simulink model "ThreeSinglePhaseDiodeRectifierSchematic"  (R2018a)
settings: Solver=VariableStepAuto  StartTime=0.0  StopTime=0.1  RelTol=1e-3
libraries: powerlib x32
settings Model: Creator=mertelmas  LastModifiedBy=mertelmas

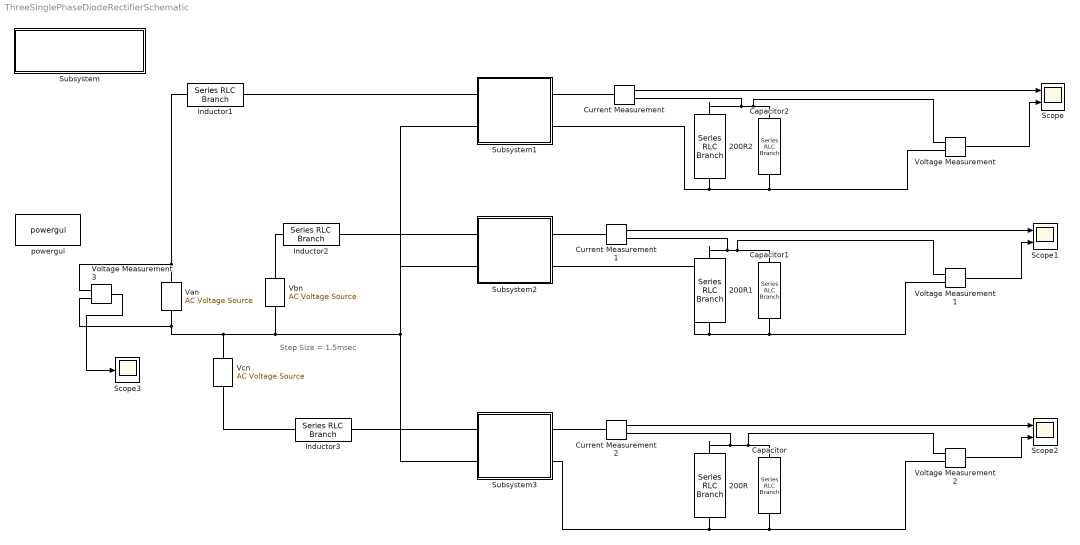
== system ThreeSinglePhaseDiodeRectifierSchematic ==
  note: Step Size = 1.5msec
  200R : powerlib/Elements/Series RLC Branch  LConnTagsString=__new0  RConnTagsString=__new0  BranchType=R  Resistance=200  Inductance=1e-3  SetiL0=off  InitialCurrent=0  Capacitance=1e-6  Setx0=off  InitialVoltage=0  Measurements=None
  200R1 : powerlib/Elements/Series RLC Branch  LConnTagsString=__new0  RConnTagsString=__new0  BranchType=R  Resistance=200  Inductance=1e-3  SetiL0=off  InitialCurrent=0  Capacitance=1e-6  Setx0=off  InitialVoltage=0  Measurements=None
  200R2 : powerlib/Elements/Series RLC Branch  LConnTagsString=__new0  RConnTagsString=__new0  BranchType=R  Resistance=200  Inductance=1e-3  SetiL0=off  InitialCurrent=0  Capacitance=1e-6  Setx0=off  InitialVoltage=0  Measurements=None
  Capacitor : powerlib/Elements/Series RLC Branch  LConnTagsString=__new0  RConnTagsString=__new0  BranchType=C  Resistance=1  Inductance=1e-3  SetiL0=off  InitialCurrent=0  Capacitance=47e-5  Setx0=off  InitialVoltage=0  Measurements=None
  Capacitor1 : powerlib/Elements/Series RLC Branch  LConnTagsString=__new0  RConnTagsString=__new0  BranchType=C  Resistance=1  Inductance=1e-3  SetiL0=off  InitialCurrent=0  Capacitance=47e-5  Setx0=off  InitialVoltage=0  Measurements=None
  Capacitor2 : powerlib/Elements/Series RLC Branch  LConnTagsString=__new0  RConnTagsString=__new0  BranchType=C  Resistance=1  Inductance=1e-3  SetiL0=off  InitialCurrent=0  Capacitance=47e-5  Setx0=off  InitialVoltage=0  Measurements=None
  Current Measurement : powerlib/Measurements/Current Measurement  PhasorSimulation=off  OutputType=Complex  PSBequivalent=0
  Current Measurement1 : powerlib/Measurements/Current Measurement  PhasorSimulation=off  OutputType=Complex  PSBequivalent=0
  Current Measurement2 : powerlib/Measurements/Current Measurement  PhasorSimulation=off  OutputType=Complex  PSBequivalent=0
  Inductor1 : powerlib/Elements/Series RLC Branch  LConnTagsString=__new0  RConnTagsString=__new0  BranchType=L  Resistance=1  Inductance=6e-4  SetiL0=off  InitialCurrent=0  Capacitance=1e-6  Setx0=off  InitialVoltage=0  Measurements=None
  Inductor2 : powerlib/Elements/Series RLC Branch  LConnTagsString=__new0  RConnTagsString=__new0  BranchType=L  Resistance=1  Inductance=6e-4  SetiL0=off  InitialCurrent=0  Capacitance=1e-6  Setx0=off  InitialVoltage=0  Measurements=None
  Inductor3 : powerlib/Elements/Series RLC Branch  LConnTagsString=__new0  RConnTagsString=__new0  BranchType=L  Resistance=1  Inductance=6e-4  SetiL0=off  InitialCurrent=0  Capacitance=1e-6  Setx0=off  InitialVoltage=0  Measurements=None
  Scope : Scope  NumInputPorts=2
  Scope1 : Scope  NumInputPorts=2
  Scope2 : Scope  NumInputPorts=2
  Scope3 : Scope
  Subsystem : Subsystem
      settings: OpenFcn=open_system('power_new_palette')
      mask Display: disp(sprintf('Open Simscape Power Systems\n(Specialized Technology)\nPalette Library'));
  Subsystem1 : Subsystem
  Subsystem2 : Subsystem
  Subsystem3 : Subsystem
  Van : powerlib/Electrical Sources/AC Voltage Source  Amplitude=325.27  Phase=0  Frequency=50  SampleTime=0  Measurements=None  BusType=swing  Pref=10e3  Qref=0  Qmin=-inf  Qmax=+inf
  Vbn : powerlib/Electrical Sources/AC Voltage Source  Amplitude=325.27  Phase=120  Frequency=50  SampleTime=0  Measurements=None  BusType=swing  Pref=10e3  Qref=0  Qmin=-inf  Qmax=+inf
  Vcn : powerlib/Electrical Sources/AC Voltage Source  Amplitude=325.27  Phase=240  Frequency=50  SampleTime=0  Measurements=None  BusType=swing  Pref=10e3  Qref=0  Qmin=-inf  Qmax=+inf
  Voltage Measurement{,1..3} (4 alike) : powerlib/Measurements/Voltage Measurement  PhasorSimulation=off  OutputType=Complex  PSBequivalent=0
  powergui : powerlib/powergui  Priority=1  SimulationMode=Continuous  SampleTime=50e-6  frequency=60  Iterations=50  frequencyindice=50  Pbase=100e6  ErrMax=1e-4  UnitsV=kV  UnitsW=MW  buscounter=0  FunctionMessages=off  echomessages=off  EnableUseOfTLC=off  CurrentSourceSwitches=off  DisableSnubberDevices=off  DisableRonSwitches=off  DisableVfSwitches=off  DisplayEquations=off  SolverType=Tustin/Backward Euler (TBE)  Interpol=off  ExternalGateDelay=off  methode=off  Ts=100  x0status=blocks  SPID=on  SwTol=0  HookPort=off  RestoreLinks=warning  ResistiveCurrentMeasurement=off  Frange=[0:2:500]  Ylog=off  Xlog=on  ShowGrid=off  save=off  variable=ZData  structure=0  ZoomFFT=off  StartTime=0.0  cycles=1  DisplayStyle=1  fundamental=60  FreqAxis=off  MaxFrequency=1000  frequencyindicesteady=1  RmsSteady=1  display=off
  wires:
  Current Measurement/1 -> Scope/1
  Current Measurement1/1 -> Scope1/1
  Current Measurement2/1 -> Scope2/1
  Voltage Measurement2/1 -> Scope2/2
  Voltage Measurement1/1 -> Scope1/2
  Voltage Measurement/1 -> Scope/2
  Voltage Measurement3/1 -> Scope3/1
  connections:
  Van/LConn1 -- Voltage Measurement3/LConn2 -- Vcn/LConn1 -- Subsystem1/LConn2 -- Subsystem2/LConn2 -- Subsystem3/LConn2 -- Vbn/LConn1
  Vcn/RConn1 -- Inductor3/LConn1
  Inductor1/LConn1 -- Voltage Measurement3/LConn1 -- Van/RConn1
  Vbn/RConn1 -- Inductor2/LConn1
  200R/LConn1 -- Current Measurement2/RConn1 -- Voltage Measurement2/LConn1 -- Capacitor/LConn1
  200R/RConn1 -- Voltage Measurement2/LConn2 -- Capacitor/RConn1 -- Subsystem3/RConn2
  200R1/LConn1 -- Current Measurement1/RConn1 -- Voltage Measurement1/LConn1 -- Capacitor1/LConn1
  200R1/RConn1 -- Voltage Measurement1/LConn2 -- Capacitor1/RConn1 -- Subsystem2/RConn2
  200R2/LConn1 -- Current Measurement/RConn1 -- Voltage Measurement/LConn1 -- Capacitor2/LConn1
  Inductor1/RConn1 -- Subsystem1/LConn1
  Inductor2/RConn1 -- Subsystem2/LConn1
  Subsystem3/LConn1 -- Inductor3/RConn1
  200R2/RConn1 -- Voltage Measurement/LConn2 -- Capacitor2/RConn1 -- Subsystem1/RConn2
  Current Measurement/LConn1 -- Subsystem1/RConn1
  Subsystem2/RConn1 -- Current Measurement1/LConn1
  Subsystem3/RConn1 -- Current Measurement2/LConn1

== system ThreeSinglePhaseDiodeRectifierSchematic/Subsystem ==

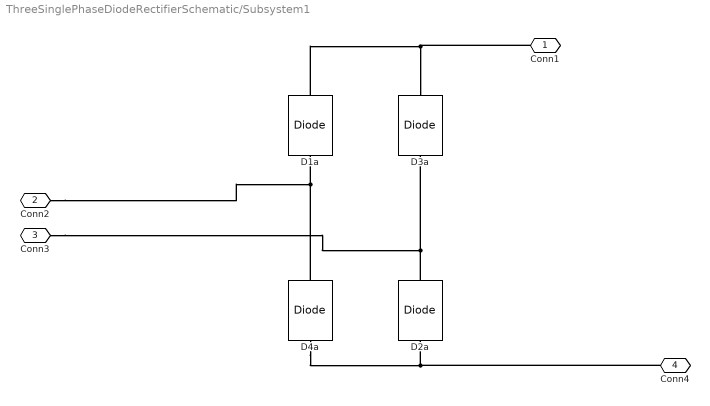
== system ThreeSinglePhaseDiodeRectifierSchematic/Subsystem1 ==
  D1a : powerlib/Power Electronics/Diode  Ron=0.001  Lon=0  Vf=0.8  IC=0  UseSnubber=0  Rs=500  Cs=250e-9  Measurements=off
  D2a : powerlib/Power Electronics/Diode  Ron=0.001  Lon=0  Vf=0.8  IC=0  UseSnubber=0  Rs=500  Cs=250e-9  Measurements=off
  D3a : powerlib/Power Electronics/Diode  Ron=0.001  Lon=0  Vf=0.8  IC=0  UseSnubber=0  Rs=500  Cs=250e-9  Measurements=off
  D4a : powerlib/Power Electronics/Diode  Ron=0.001  Lon=0  Vf=0.8  IC=0  UseSnubber=0  Rs=500  Cs=250e-9  Measurements=off
  Conn1 : PMIOPort  Side=Right
  Conn2 : PMIOPort  Port=2  Side=Left
  Conn3 : PMIOPort  Port=3  Side=Left
  Conn4 : PMIOPort  Port=4  Side=Right
  connections:
  D1a/RConn1 -- D3a/RConn1 -- Conn1/RConn1
  D2a/RConn1 -- D3a/LConn1 -- Conn3/RConn1
  D4a/LConn1 -- D2a/LConn1 -- Conn4/RConn1
  D4a/RConn1 -- D1a/LConn1 -- Conn2/RConn1

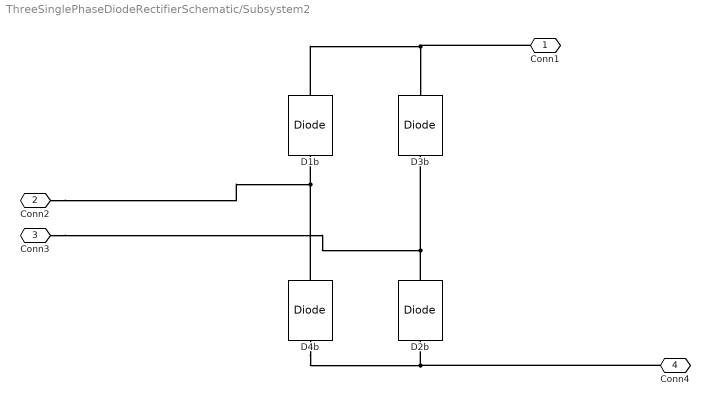
== system ThreeSinglePhaseDiodeRectifierSchematic/Subsystem2 ==
  D1b : powerlib/Power Electronics/Diode  Ron=0.001  Lon=0  Vf=0.8  IC=0  UseSnubber=0  Rs=500  Cs=250e-9  Measurements=off
  D2b : powerlib/Power Electronics/Diode  Ron=0.001  Lon=0  Vf=0.8  IC=0  UseSnubber=0  Rs=500  Cs=250e-9  Measurements=off
  D3b : powerlib/Power Electronics/Diode  Ron=0.001  Lon=0  Vf=0.8  IC=0  UseSnubber=0  Rs=500  Cs=250e-9  Measurements=off
  D4b : powerlib/Power Electronics/Diode  Ron=0.001  Lon=0  Vf=0.8  IC=0  UseSnubber=0  Rs=500  Cs=250e-9  Measurements=off
  Conn1 : PMIOPort  Side=Right
  Conn2 : PMIOPort  Port=2  Side=Left
  Conn3 : PMIOPort  Port=3  Side=Left
  Conn4 : PMIOPort  Port=4  Side=Right
  connections:
  D1b/RConn1 -- D3b/RConn1 -- Conn1/RConn1
  D2b/RConn1 -- D3b/LConn1 -- Conn3/RConn1
  D4b/LConn1 -- D2b/LConn1 -- Conn4/RConn1
  D4b/RConn1 -- D1b/LConn1 -- Conn2/RConn1

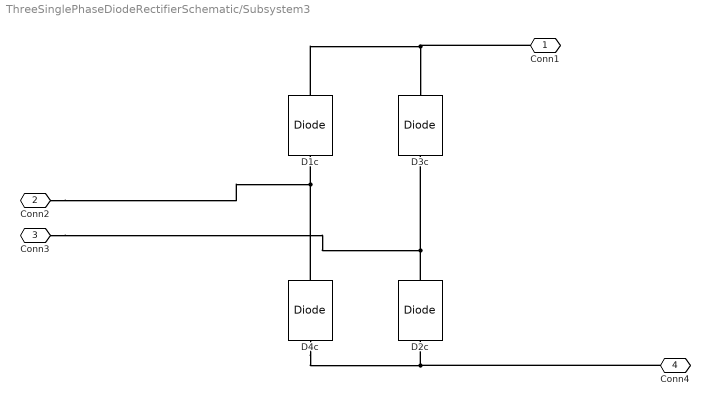
== system ThreeSinglePhaseDiodeRectifierSchematic/Subsystem3 ==
  D1c : powerlib/Power Electronics/Diode  Ron=0.001  Lon=0  Vf=0.8  IC=0  UseSnubber=0  Rs=500  Cs=250e-9  Measurements=off
  D2c : powerlib/Power Electronics/Diode  Ron=0.001  Lon=0  Vf=0.8  IC=0  UseSnubber=0  Rs=500  Cs=250e-9  Measurements=off
  D3c : powerlib/Power Electronics/Diode  Ron=0.001  Lon=0  Vf=0.8  IC=0  UseSnubber=0  Rs=500  Cs=250e-9  Measurements=off
  D4c : powerlib/Power Electronics/Diode  Ron=0.001  Lon=0  Vf=0.8  IC=0  UseSnubber=0  Rs=500  Cs=250e-9  Measurements=off
  Conn1 : PMIOPort  Side=Right
  Conn2 : PMIOPort  Port=2  Side=Left
  Conn3 : PMIOPort  Port=3  Side=Left
  Conn4 : PMIOPort  Port=4  Side=Right
  connections:
  D1c/RConn1 -- D3c/RConn1 -- Conn1/RConn1
  D2c/RConn1 -- D3c/LConn1 -- Conn3/RConn1
  D4c/LConn1 -- D2c/LConn1 -- Conn4/RConn1
  D4c/RConn1 -- D1c/LConn1 -- Conn2/RConn1
